simulink model "Cinematica_Inversa_Jacobiana_Traspuesta"  (R2015a)
settings: Solver=ode45  StartTime=0.0  StopTime=2  RelTol=1e-3
values from neighbouring files (symbols this model uses):
  dif_t = in(9)    [Euler.m]    (also in rob_sic.m = 0.001)
settings Model: Creator=TRIANOSAURIO  LastModifiedBy=TRIANOSAURIO

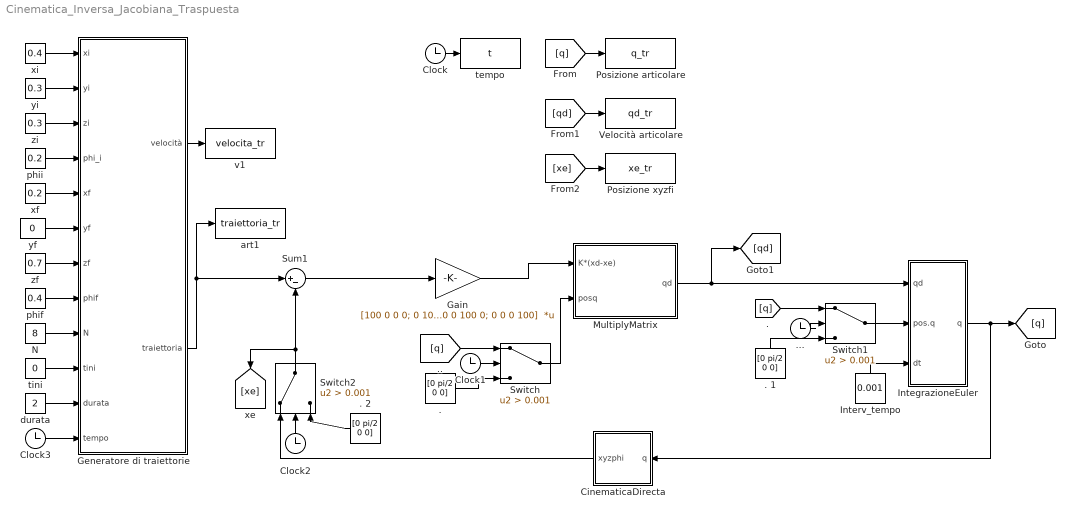
== system Cinematica_Inversa_Jacobiana_Traspuesta ==
  ". " : Constant  Value=[0 pi/2 0 0]
  . 1 : Constant  Value=[0 pi/2 0 0]
  . 2 : Constant  Value=[0 pi/2 0 0]
  "... " : Clock
  CinematicaDirecta : Subsystem
  Clock{,1..3} (4 alike) : Clock
  Gain : Gain  Gain=[100 0 0 0; 0 100 0 0; 0 0 100 0; 0 0 0 100]  Multiplication=Matrix(K*u)
  Generatore di traiettorie : Subsystem
  IntegrazioneEuler : Subsystem
  Interv_tempo : Constant  Value=0.001
  MultiplyMatrix : Subsystem
  N : Constant  Value=8
  Posizione articolare : ToWorkspace  VariableName=q_tr  SampleTime=dif_t
  "Posizione xyzfi " : ToWorkspace  VariableName=xe_tr  SampleTime=dif_t
  Sum1 : Sum  Inputs=|+-
  Switch : Switch  Criteria=u2 > Threshold  Threshold=0.001
  Switch1 : Switch  Criteria=u2 > Threshold  Threshold=0.001
  Switch2 : Switch  Criteria=u2 > Threshold  Threshold=0.001
  Velocità articolare : ToWorkspace  VariableName=qd_tr  SampleTime=dif_t
  art1 : ToWorkspace  VariableName=traiettoria_tr  SampleTime=dif_t
  durata : Constant  Value=2
  phif : Constant  Value=0.4
  phii : Constant  Value=0.2
  tempo : ToWorkspace  VariableName=t  SampleTime=0.001
  tini : Constant  Value=0
  v1 : ToWorkspace  VariableName=velocita_tr  SampleTime=dif_t
  xf : Constant  Value=0.2
  xi : Constant  Value=0.4
  yf : Constant  Value=0
  yi : Constant  Value=0.3
  zf : Constant  Value=0.7
  zi : Constant  Value=0.3
  wires:
  Sum1/1 -> Gain/1
  Clock/1 -> tempo/1
  IntegrazioneEuler/1(q) -> CinematicaDirecta/1(q), [q]
  [q] -> Posizione articolare/1
  Gain/1 -> MultiplyMatrix/1(K*(xd-xe))
  MultiplyMatrix/1(qd) -> [qd], IntegrazioneEuler/1(qd)
  Interv_tempo/1 -> IntegrazioneEuler/3(dt)
  Switch/1 -> MultiplyMatrix/2(posq)
  Clock1/1 -> Switch/2
  [q] -> Switch1/1
  Switch1/1 -> IntegrazioneEuler/2(pos.q)
  "... "/1 -> Switch1/2
  . 1/1 -> Switch1/3
  [q] -> Switch/1
  ". "/1 -> Switch/3
  Switch2/1 -> Sum1/2, [xe]
  CinematicaDirecta/1(xyzphi) -> Switch2/1
  Clock2/1 -> Switch2/2
  . 2/1 -> Switch2/3
  [qd] -> Velocità articolare/1
  [xe] -> "Posizione xyzfi "/1
  xi/1 -> Generatore di traiettorie/1(xi)
  yi/1 -> Generatore di traiettorie/2(yi)
  zi/1 -> Generatore di traiettorie/3(zi)
  phii/1 -> Generatore di traiettorie/4(phi_i)
  xf/1 -> Generatore di traiettorie/5(xf)
  yf/1 -> Generatore di traiettorie/6(yf)
  zf/1 -> Generatore di traiettorie/7(zf)
  phif/1 -> Generatore di traiettorie/8(phif)
  N/1 -> Generatore di traiettorie/9(N)
  tini/1 -> Generatore di traiettorie/10(tini)
  durata/1 -> Generatore di traiettorie/11(durata)
  Clock3/1 -> Generatore di traiettorie/12(tempo)
  Generatore di traiettorie/2("traiettoria ") -> Sum1/1, art1/1
  Generatore di traiettorie/1(velocità) -> v1/1

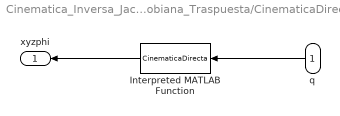
== system Cinematica_Inversa_Jacobiana_Traspuesta/CinematicaDirecta ==
  q : Inport
  Interpreted MATLAB Function : MATLABFcn  MATLABFcn=CinematicaDirecta
  xyzphi : Outport
  wires:
  q/1 -> Interpreted MATLAB Function/1
  Interpreted MATLAB Function/1 -> xyzphi/1

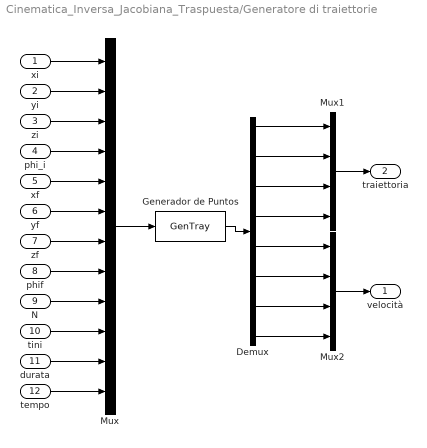
== system Cinematica_Inversa_Jacobiana_Traspuesta/Generatore di traiettorie ==
  xi : Inport
  yi : Inport  Port=2
  zi : Inport  Port=3
  phi_i : Inport  Port=4
  xf : Inport  Port=5
  yf : Inport  Port=6
  zf : Inport  Port=7
  phif : Inport  Port=8
  N : Inport  Port=9
  tini : Inport  Port=10
  durata : Inport  Port=11
  tempo : Inport  Port=12
  Demux : Demux  Outputs=8
  Generador de Puntos : MATLABFcn  MATLABFcn=GenTray  OutputDimensions=8
  Mux : Mux  Inputs=12
  Mux1 : Mux
  Mux2 : Mux
  velocità : Outport
  "traiettoria " : Outport  Port=2
  wires:
  Mux/1 -> Generador de Puntos/1
  xi/1 -> Mux/1
  yi/1 -> Mux/2
  zi/1 -> Mux/3
  phi_i/1 -> Mux/4
  xf/1 -> Mux/5
  yf/1 -> Mux/6
  zf/1 -> Mux/7
  phif/1 -> Mux/8
  N/1 -> Mux/9
  tini/1 -> Mux/10
  durata/1 -> Mux/11
  tempo/1 -> Mux/12
  Generador de Puntos/1 -> Demux/1
  Mux1/1 -> "traiettoria "/1
  Demux/1 -> Mux1/1
  Demux/2 -> Mux1/2
  Demux/3 -> Mux1/3
  Demux/4 -> Mux1/4
  Demux/5 -> Mux2/1
  Demux/6 -> Mux2/2
  Demux/7 -> Mux2/3
  Demux/8 -> Mux2/4
  Mux2/1 -> velocità/1

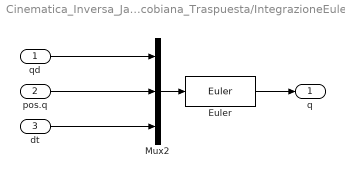
== system Cinematica_Inversa_Jacobiana_Traspuesta/IntegrazioneEuler ==
  qd : Inport
  pos.q : Inport  Port=2
  dt : Inport  Port=3
  Euler : MATLABFcn  MATLABFcn=Euler
  Mux2 : Mux  Inputs=3
  q : Outport
  wires:
  Euler/1 -> q/1
  qd/1 -> Mux2/1
  Mux2/1 -> Euler/1
  pos.q/1 -> Mux2/2
  dt/1 -> Mux2/3

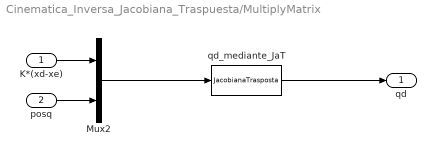
== system Cinematica_Inversa_Jacobiana_Traspuesta/MultiplyMatrix ==
  K*(xd-xe) : Inport
  posq : Inport  Port=2
  Mux2 : Mux  Inputs=2
  qd_mediante_JaT : MATLABFcn  MATLABFcn=JacobianaTrasposta
  qd : Outport
  wires:
  qd_mediante_JaT/1 -> qd/1
  Mux2/1 -> qd_mediante_JaT/1
  K*(xd-xe)/1 -> Mux2/1
  posq/1 -> Mux2/2
